simulink model "k1visetmy"  (Simulink 8.6)
settings: Solver=ode45  StartTime=0.0  StopTime=10.0  RelTol=1e-3
libraries: cdsCDI64 x10, cdsCDO64 x10, BIO_CD_DECODE_MASTER x10, BIO_CD_ENCODE_MASTER x9, cdsIPCx x5, dac x3, cdsEpicsOut x3, cdsBit2Word x2, cdsAdcx0 x1, cdsAdcx1 x1, cdsCDO32 x1, TYPEA_MASTER x1
settings Model: Creator=controls  LastModifiedBy=controls
settings DataIOCC: SignalLoggingSaveFormat=Dataset
settings OptimizationCC: ExpressionDepthLimit=128
settings DebuggingCC: UnderspecifiedInitializationDetection=Simplified  MergeDetectMultiDrivingBlocksExec=error  SolverPrmCheckMsg=none  FcnCallInpInsideContextMsg=EnableAllAsError  StateNameClashWarn=none
settings GRTTargetCC: CombineOutputUpdateFcns=on  GRTInterface=off

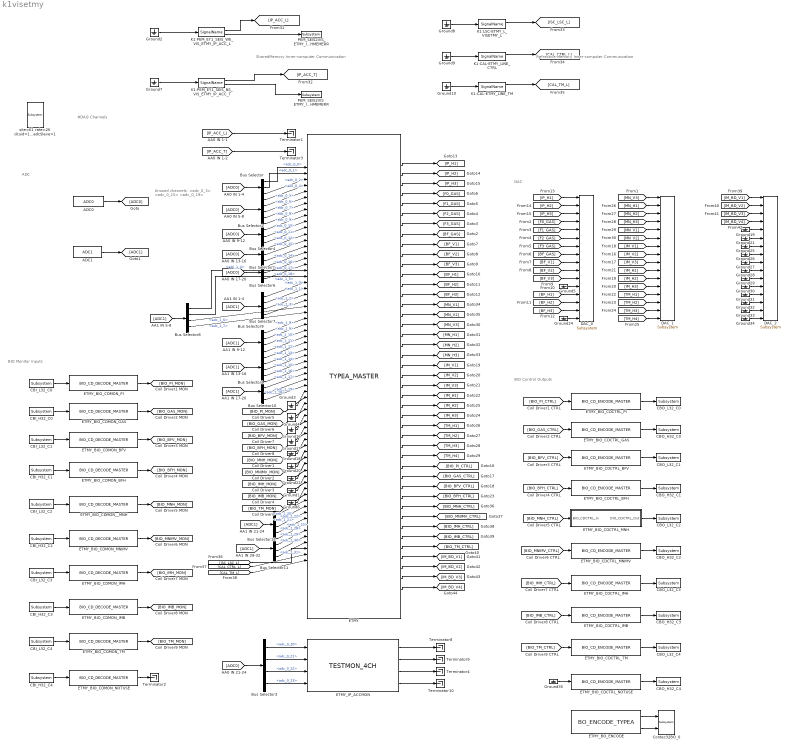
== system k1visetmy ==
  note: Unused channels:
      | <adc_0_3>
      | <adc_0_15>
      | <adc_0_19>
  note: #DAQ Channels
  note: BIO Monitor Inputs
  note: BIO Control Outputs
  note: DAC
  note: ADC
  note: SharedMemory
      | Inner-computer Communication
  note: Refrective Memory
      | Inner-computer Communication
  ADC0 : cdsAdcx0/ADC0  Tag=cdsAdc  Description=|
      | type-GSC_16AI64SSA
      | card_num=0
      settings: AttributesFormatString=%<Description>\n%<Tag>
  ADC1 : cdsAdcx1/ADC1  Tag=cdsAdc  Description=|
      | type-GSC_16AI64SSA
      | card_num=1
      settings: AttributesFormatString=%<Description>\n%<Tag>
  Bus Selector : BusSelector  OutputSignals=adc_0_0,adc_0_1,adc_0_2
  Bus Selector1 : BusSelector  OutputSignals=adc_1_12,adc_1_13,adc_1_14,adc_1_15
  Bus Selector10 : BusSelector  OutputSignals=adc_1_16,adc_1_17,adc_1_18,adc_1_19
  Bus Selector11 : BusSelector  OutputSignals=adc_1_28,adc_1_29,adc_1_30,adc_1_31
  Bus Selector12 : BusSelector  OutputSignals=adc_1_20,adc_1_21,adc_1_22,adc_1_23
  Bus Selector2 : BusSelector  OutputSignals=adc_0_4,adc_0_5,adc_0_6,adc_0_7
  Bus Selector3 : BusSelector  OutputSignals=adc_0_20,adc_0_21,adc_0_22,adc_0_23
  Bus Selector4 : BusSelector  OutputSignals=adc_0_8,adc_0_9,adc_0_10,adc_0_11
  Bus Selector5 : BusSelector  OutputSignals=adc_0_12,adc_0_15,adc_0_14
  Bus Selector6 : BusSelector  OutputSignals=adc_0_16,adc_0_17,adc_0_18
  Bus Selector7 : BusSelector  OutputSignals=adc_1_0,adc_1_1,adc_1_2,adc_1_3
  Bus Selector8 : BusSelector  OutputSignals=adc_1_4,adc_1_5,adc_1_6,adc_1_7
  Bus Selector9 : BusSelector  OutputSignals=adc_1_8,adc_1_9,adc_1_10,adc_1_11
  CBI_H32_C0 : cdsCDI64/Subsystem  Tag=cdsCDI64  Description=card_num=1
      settings: AttributesFormatString=%<Tag>\n%<Description>
  CBI_H32_C1 : cdsCDI64/Subsystem  Tag=cdsCDI64  Description=card_num=3
      settings: AttributesFormatString=%<Tag>\n%<Description>
  CBI_H32_C2 : cdsCDI64/Subsystem  Tag=cdsCDI64  Description=card_num=5
      settings: AttributesFormatString=%<Tag>\n%<Description>
  CBI_H32_C3 : cdsCDI64/Subsystem  Tag=cdsCDI64  Description=card_num=7
      settings: AttributesFormatString=%<Tag>\n%<Description>
  CBI_H32_C4 : cdsCDI64/Subsystem  Tag=cdsCDI64  Description=card_num=9
      settings: AttributesFormatString=%<Tag>\n%<Description>
  CBI_L32_C0 : cdsCDI64/Subsystem  Tag=cdsCDI64  Description=card_num=0
      settings: AttributesFormatString=%<Tag>\n%<Description>
  CBI_L32_C1 : cdsCDI64/Subsystem  Tag=cdsCDI64  Description=card_num=2
      settings: AttributesFormatString=%<Tag>\n%<Description>
  CBI_L32_C2 : cdsCDI64/Subsystem  Tag=cdsCDI64  Description=card_num=4
      settings: AttributesFormatString=%<Tag>\n%<Description>
  CBI_L32_C3 : cdsCDI64/Subsystem  Tag=cdsCDI64  Description=card_num=6
      settings: AttributesFormatString=%<Tag>\n%<Description>
  CBI_L32_C4 : cdsCDI64/Subsystem  Tag=cdsCDI64  Description=card_num=8
      settings: AttributesFormatString=%<Tag>\n%<Description>
  CBO_H32_C0 : cdsCDO64/Subsystem  Tag=cdsCDO64  Description=card_num=1
      settings: AttributesFormatString=%<Tag>\n%<Description>
  CBO_H32_C1 : cdsCDO64/Subsystem  Tag=cdsCDO64  Description=card_num=3
      settings: AttributesFormatString=%<Tag>\n%<Description>
  CBO_H32_C2 : cdsCDO64/Subsystem  Tag=cdsCDO64  Description=card_num=5
      settings: AttributesFormatString=%<Tag>\n%<Description>
  CBO_H32_C3 : cdsCDO64/Subsystem  Tag=cdsCDO64  Description=card_num=7
      settings: AttributesFormatString=%<Tag>\n%<Description>
  CBO_H32_C4 : cdsCDO64/Subsystem  Tag=cdsCDO64  Description=card_num=9
      settings: AttributesFormatString=%<Tag>\n%<Description>
  CBO_L32_C0 : cdsCDO64/Subsystem  Tag=cdsCDO64  Description=card_num=0
      settings: AttributesFormatString=%<Tag>\n%<Description>
  CBO_L32_C1 : cdsCDO64/Subsystem  Tag=cdsCDO64  Description=card_num=2
      settings: AttributesFormatString=%<Tag>\n%<Description>
  CBO_L32_C2 : cdsCDO64/Subsystem  Tag=cdsCDO64  Description=card_num=4
      settings: AttributesFormatString=%<Tag>\n%<Description>
  CBO_L32_C3 : cdsCDO64/Subsystem  Tag=cdsCDO64  Description=card_num=6
      settings: AttributesFormatString=%<Tag>\n%<Description>
  CBO_L32_C4 : cdsCDO64/Subsystem  Tag=cdsCDO64  Description=card_num=8
      settings: AttributesFormatString=%<Tag>\n%<Description>
  Contec32BO_0 : cdsCDO32/Subsystem  Tag=cdsCDO32  Description=Contec32 bit binary output module driver
      settings: AttributesFormatString=%<Tag>
  DAC_0 : dac/Subsystem  Description=|
      | type=GSC_16AO16,
      | card_num=0
      settings: AttributesFormatString=%<Description>
  DAC_1 : dac/Subsystem  Description=|
      | type=GSC_16AO16,
      | card_num=1
      settings: AttributesFormatString=%<Description>
  DAC_2 : dac/Subsystem  Description=|
      | type=GSC_16AO16,
      | card_num=2
      settings: AttributesFormatString=%<Description>
  ETMY : TYPEA_MASTER/TYPEA_MASTER
  ETMY_BIO_CDCTRL_BFH : BIO_CD_ENCODE_MASTER/BIO_CD_ENCODE_MASTER
  ETMY_BIO_CDCTRL_BFV : BIO_CD_ENCODE_MASTER/BIO_CD_ENCODE_MASTER
  ETMY_BIO_CDCTRL_GAS : BIO_CD_ENCODE_MASTER/BIO_CD_ENCODE_MASTER
  ETMY_BIO_CDCTRL_IMB : BIO_CD_ENCODE_MASTER/BIO_CD_ENCODE_MASTER
  ETMY_BIO_CDCTRL_IMH : BIO_CD_ENCODE_MASTER/BIO_CD_ENCODE_MASTER
  ETMY_BIO_CDCTRL_MNH : Subsystem
  ETMY_BIO_CDCTRL_MNIMV : BIO_CD_ENCODE_MASTER/BIO_CD_ENCODE_MASTER
  ETMY_BIO_CDCTRL_NOTUSE : BIO_CD_ENCODE_MASTER/BIO_CD_ENCODE_MASTER
  ETMY_BIO_CDCTRL_PI : BIO_CD_ENCODE_MASTER/BIO_CD_ENCODE_MASTER
  ETMY_BIO_CDCTRL_TM : BIO_CD_ENCODE_MASTER/BIO_CD_ENCODE_MASTER
  ETMY_BIO_CDMON_BFH : BIO_CD_DECODE_MASTER/BIO_CD_DECODE_MASTER
  ETMY_BIO_CDMON_BFV : BIO_CD_DECODE_MASTER/BIO_CD_DECODE_MASTER
  ETMY_BIO_CDMON_GAS : BIO_CD_DECODE_MASTER/BIO_CD_DECODE_MASTER
  ETMY_BIO_CDMON_IMB : BIO_CD_DECODE_MASTER/BIO_CD_DECODE_MASTER
  ETMY_BIO_CDMON_IMH : BIO_CD_DECODE_MASTER/BIO_CD_DECODE_MASTER
  ETMY_BIO_CDMON_MNIMV : BIO_CD_DECODE_MASTER/BIO_CD_DECODE_MASTER
  ETMY_BIO_CDMON_NOTUSE : BIO_CD_DECODE_MASTER/BIO_CD_DECODE_MASTER
  ETMY_BIO_CDMON_PI : BIO_CD_DECODE_MASTER/BIO_CD_DECODE_MASTER
  ETMY_BIO_CDMON_TM : BIO_CD_DECODE_MASTER/BIO_CD_DECODE_MASTER
  ETMY_BIO_CDMON__MNH : BIO_CD_DECODE_MASTER/BIO_CD_DECODE_MASTER
  ETMY_BO_ENCODE : BO_TYPEA_MASTER/BO_ENCODE_TYPEA
  ETMY_IP_ACCMON : TESTMON_4CH_MASTER/TESTMON_4CH
  Ground{1..10,16..22,24..35} (29 alike) : Ground
  K1:CAL-ETMY_LINE_CTRL : cdsIPCx/SignalName  Tag=cdsIPCx_RFM  Description=card=0
      settings: AttributesFormatString=%<Description>\n%<Tag>
  K1:CAL-ETMY_LINE_TM : cdsIPCx/SignalName  Tag=cdsIPCx_RFM  Description=card=0
      settings: AttributesFormatString=%<Description>\n%<Tag>
  K1:LSC-ETMY_L_VISETMY_L : cdsIPCx/SignalName  Tag=cdsIPCx_RFM  Description=card=0
      settings: AttributesFormatString=%<Description>\n%<Tag>
  K1:PEM_EY1_SEIS_NS_VIS_ETMY_IP_ACC_T : cdsIPCx/SignalName  Tag=cdsIPCx_SHMEM  Description=Inter-Process Communication via Shared memory.
      settings: AttributesFormatString=%<Tag>
  K1:PEM_EY1_SEIS_WE_VIS_ETMY_IP_ACC_L : cdsIPCx/SignalName  Tag=cdsIPCx_SHMEM  Description=Inter-Process Communication via Shared memory.
      settings: AttributesFormatString=%<Tag>
  PEM_SEIS2VIS_ETMY_IP_ACC_L_SHMEMERR : cdsEpicsOut/Subsystem  Tag=cdsEpicsOutput  Description=|
      | Purpose:                                          
      | Output a FE signal to an EPICS channel.           
      |                                                   
      | Operation:                                        
      | Takes input value and passes it to EPICS record.  
      |                                                   
      | Usage:                                            
      | Name the part with the desired EPICS rrecord name.
      settings: AttributesFormatString=%<Tag>
  PEM_SEIS2VIS_ETMY_IP_ACC_T_SHMEMERR : cdsEpicsOut/Subsystem  Tag=cdsEpicsOutput  Description=|
      | Purpose:                                          
      | Output a FE signal to an EPICS channel.           
      |                                                   
      | Operation:                                        
      | Takes input value and passes it to EPICS record.  
      |                                                   
      | Usage:                                            
      | Name the part with the desired EPICS rrecord name.
      settings: AttributesFormatString=%<Tag>
  Terminator{1..4,8..10} (7 alike) : Terminator
  site=K1 rate=2K dcuid=106 host=k1ey1 specific_cpu=3 adcSlave=1 : cdsParameters/Subsystem  Tag=cdsParameters  Description=|
      | Purpose:                                                                                                                                                                                                                                
      | Provide system parameters to the FE code generator to properly configure the generated EPICS names, rep rate of the FE controller, and the Data Acquisition node ID for proper storage of data from this FE controller.                 
      |                                                                                                                                                                                                                                         
      | Useage:                                                                                                                                                                                                                                 
      | The part NAME field is used to identify the FE parameters. It must be of the form:                                                                                                                                                      
      | site=                                                                                                                                                                                                                                   
      | rate=                                                                                                                                                                                                                                   
      | dcuid=                                                                                                                                                                                                                                  
      |                                                                                                                                                                                                                                         
      | Where:                                                                                                                                                                                                                                  
      | site= argument may be H1, H2, L1, M1, G1, either as a single argument or multiple, for example site=H1,H2. These are the only names allowed. These will become the first two characters of all EPICS and signal names (for example G1:).
      |                                                                                                                                                                                                                                         
      | rate= may be 2K, 16K, 32K, or 64K                                                                                                                                                                                                       
      |                                                                                                                                                                                                                                         
      | dcuid= is site specific ie it must be unique at each site.
      settings: AttributesFormatString=%<Tag>
  wires:
  ADC0/1 -> [ADC0]
  ADC1/1 -> [ADC1]
  [ADC0] -> Bus Selector/1
  [ADC0] -> Bus Selector2/1
  [ADC0] -> Bus Selector4/1
  [ADC0] -> Bus Selector5/1
  Bus Selector5/1 -> ETMY/12  "<adc_0_12>"
  Bus Selector5/3 -> ETMY/14  "<adc_0_14>"
  Bus Selector5/2 -> ETMY/13  "<adc_0_15>"
  [ADC0] -> Bus Selector6/1
  Bus Selector6/1 -> ETMY/15  "<adc_0_16>"
  Bus Selector6/2 -> ETMY/16  "<adc_0_17>"
  ETMY/10 -> [BF_V2]
  ETMY/11 -> [BF_V3]
  ETMY/12 -> [BF_H1]
  ETMY/13 -> [BF_H2]
  ETMY/14 -> [BF_H3]
  [BF_H2] -> DAC_0/14
  [BF_V3] -> DAC_0/11
  [BF_H3] -> DAC_0/15
  [BF_V1] -> DAC_0/9
  [BF_H1] -> DAC_0/13
  [BF_V2] -> DAC_0/10
  CBI_H32_C0/1 -> ETMY_BIO_CDMON_GAS/1
  CBI_L32_C1/1 -> ETMY_BIO_CDMON_BFV/1
  CBI_L32_C0/1 -> ETMY_BIO_CDMON_PI/1
  CBI_H32_C1/1 -> ETMY_BIO_CDMON_BFH/1
  ETMY_BIO_CDCTRL_BFH/1 -> CBO_H32_C1/1
  ETMY_BIO_CDCTRL_PI/1 -> CBO_L32_C0/1
  ETMY_BIO_CDCTRL_GAS/1 -> CBO_H32_C0/1
  ETMY_BIO_CDCTRL_BFV/1 -> CBO_L32_C1/1
  [BIO_PI_CTRL] -> ETMY_BIO_CDCTRL_PI/1
  [BIO_GAS_CTRL] -> ETMY_BIO_CDCTRL_GAS/1
  [BIO_BFV_CTRL] -> ETMY_BIO_CDCTRL_BFV/1
  ETMY_BIO_CDMON_PI/1 -> [BIO_PI_MON]
  ETMY_BIO_CDMON_GAS/1 -> [BIO_GAS_MON]
  ETMY_BIO_CDMON_BFH/1 -> [BIO_BFH_MON]
  ETMY_BIO_CDMON_BFV/1 -> [BIO_BFV_MON]
  [BIO_BFH_CTRL] -> ETMY_BIO_CDCTRL_BFH/1
  Bus Selector/1 -> ETMY/1  "<adc_0_0>"
  Bus Selector/2 -> ETMY/2  "<adc_0_1>"
  Bus Selector/3 -> ETMY/3  "<adc_0_2>"
  Bus Selector2/1 -> ETMY/4  "<adc_0_4>"
  Bus Selector2/2 -> ETMY/5  "<adc_0_5>"
  Bus Selector2/3 -> ETMY/6  "<adc_0_6>"
  Bus Selector2/4 -> ETMY/7  "<adc_0_7>"
  Bus Selector4/1 -> ETMY/8  "<adc_0_8>"
  Bus Selector4/2 -> ETMY/9  "<adc_0_9>"
  Bus Selector4/3 -> ETMY/10  "<adc_0_10>"
  Bus Selector4/4 -> ETMY/11  "<adc_0_11>"
  [IP_H1] -> DAC_0/1
  [IP_H2] -> DAC_0/2
  [IP_H3] -> DAC_0/3
  [F0_GAS] -> DAC_0/4
  [F1_GAS] -> DAC_0/5
  [F2_GAS] -> DAC_0/6
  [F3_GAS] -> DAC_0/7
  [BF_GAS] -> DAC_0/8
  [ADC0] -> Bus Selector3/1
  Bus Selector3/2 -> ETMY_IP_ACCMON/2  "<adc_0_21>"
  Bus Selector3/1 -> ETMY_IP_ACCMON/1  "<adc_0_20>"
  Bus Selector3/3 -> ETMY_IP_ACCMON/3  "<adc_0_22>"
  Bus Selector3/4 -> ETMY_IP_ACCMON/4  "<adc_0_23>"
  ETMY_IP_ACCMON/3 -> Terminator4/1
  ETMY_IP_ACCMON/4 -> Terminator10/1
  ETMY_IP_ACCMON/1 -> Terminator8/1
  ETMY_IP_ACCMON/2 -> Terminator9/1
  Bus Selector6/3 -> ETMY/17  "<adc_0_18>"
  Ground5/1 -> DAC_0/12
  Ground24/1 -> DAC_0/16
  [ADC1] -> Bus Selector7/1
  [ADC1] -> Bus Selector8/1
  [ADC1] -> Bus Selector9/1
  [IM_H2] -> DAC_1/11
  [IM_H1] -> DAC_1/10
  [IM_V1] -> DAC_1/7
  [IM_V2] -> DAC_1/8
  [IM_V3] -> DAC_1/9
  [TM_H3] -> DAC_1/15
  [TM_H2] -> DAC_1/14
  [TM_H1] -> DAC_1/13
  [TM_H4] -> DAC_1/16
  [IM_H3] -> DAC_1/12
  [MN_V3] -> DAC_1/1
  [MN_H1] -> DAC_1/2
  [MN_H2] -> DAC_1/3
  [MN_H3] -> DAC_1/4
  [MN_V1] -> DAC_1/5
  [MN_V2] -> DAC_1/6
  [ADC1] -> Bus Selector1/1
  [ADC1] -> Bus Selector10/1
  [BIO_PI_MON] -> ETMY/39
  [BIO_GAS_MON] -> ETMY/41
  [BIO_BFV_MON] -> ETMY/43
  [BIO_BFH_MON] -> ETMY/45
  Ground3/1 -> ETMY/38
  Ground4/1 -> ETMY/40
  Ground16/1 -> ETMY/42
  Ground17/1 -> ETMY/44
  Ground18/1 -> ETMY/46
  [BIO_MNH_MON] -> ETMY/47
  Ground20/1 -> ETMY/48
  [BIO_MNIMV_MON] -> ETMY/49
  Ground22/1 -> ETMY/50
  [BIO_IMH_MON] -> ETMY/51
  Bus Selector8/1 -> ETMY/18  "<adc_1_4>"
  Bus Selector8/2 -> ETMY/19  "<adc_1_5>"
  Bus Selector8/3 -> ETMY/24  "<adc_1_6>"
  Bus Selector8/4 -> ETMY/25  "<adc_1_7>"
  Bus Selector7/1 -> ETMY/20  "<adc_1_0>"
  Bus Selector7/2 -> ETMY/21  "<adc_1_1>"
  Bus Selector7/3 -> ETMY/22  "<adc_1_2>"
  Bus Selector7/4 -> ETMY/23  "<adc_1_3>"
  Bus Selector9/1 -> ETMY/26  "<adc_1_8>"
  Bus Selector9/2 -> ETMY/27  "<adc_1_9>"
  Bus Selector9/3 -> ETMY/28  "<adc_1_10>"
  Bus Selector9/4 -> ETMY/29  "<adc_1_11>"
  Bus Selector1/1 -> ETMY/30  "<adc_1_12>"
  Bus Selector1/2 -> ETMY/31  "<adc_1_13>"
  Bus Selector1/3 -> ETMY/32  "<adc_1_14>"
  Bus Selector1/4 -> ETMY/33  "<adc_1_15>"
  Bus Selector10/1 -> ETMY/34  "<adc_1_16>"
  Bus Selector10/2 -> ETMY/35  "<adc_1_17>"
  Bus Selector10/3 -> ETMY/36  "<adc_1_18>"
  Bus Selector10/4 -> ETMY/37  "<adc_1_19>"
  Ground1/1 -> ETMY/52
  Ground6/1 -> ETMY/54
  [BIO_IMB_MON] -> ETMY/53
  [BIO_TM_MON] -> ETMY/55
  ETMY/15 -> [MN_V1]
  ETMY/16 -> [MN_V2]
  ETMY/17 -> [MN_V3]
  ETMY/19 -> [MN_H2]
  ETMY/18 -> [MN_H1]
  ETMY/21 -> [IM_V1]
  ETMY/20 -> [MN_H3]
  ETMY/22 -> [IM_V2]
  ETMY/23 -> [IM_V3]
  ETMY/25 -> [IM_H2]
  ETMY/24 -> [IM_H1]
  ETMY/27 -> [TM_H1]
  ETMY/26 -> [IM_H3]
  ETMY/28 -> [TM_H2]
  ETMY/30 -> [TM_H4]
  ETMY/29 -> [TM_H3]
  ETMY/31 -> [BIO_PI_CTRL]
  ETMY/32 -> [BIO_GAS_CTRL]
  ETMY/33 -> [BIO_BFV_CTRL]
  ETMY/37 -> [BIO_IMH_CTRL]
  ETMY/34 -> [BIO_BFH_CTRL]
  ETMY/36 -> [BIO_MNIMV_CTRL]
  ETMY/35 -> [BIO_MNH_CTRL]
  ETMY/39 -> [BIO_TM_CTRL]
  ETMY/38 -> [BIO_IMB_CTRL]
  ETMY_BIO_CDCTRL_MNH/1(DIO_CDCTRL_Out) -> CBO_L32_C2/1
  ETMY_BIO_CDCTRL_MNIMV/1 -> CBO_H32_C2/1
  [BIO_MNH_CTRL] -> ETMY_BIO_CDCTRL_MNH/1(BIO_CDCTRL_In)
  [BIO_MNIMV_CTRL] -> ETMY_BIO_CDCTRL_MNIMV/1
  CBI_L32_C2/1 -> ETMY_BIO_CDMON__MNH/1
  CBI_H32_C2/1 -> ETMY_BIO_CDMON_MNIMV/1
  ETMY_BIO_CDMON__MNH/1 -> [BIO_MNH_MON]
  ETMY_BIO_CDMON_MNIMV/1 -> [BIO_MNIMV_MON]
  Ground19/1 -> DAC_2/5
  Ground21/1 -> DAC_2/6
  Ground25/1 -> DAC_2/7
  Ground26/1 -> DAC_2/8
  Ground27/1 -> DAC_2/9
  Ground28/1 -> DAC_2/10
  Ground29/1 -> DAC_2/11
  Ground30/1 -> DAC_2/12
  Ground31/1 -> DAC_2/13
  Ground32/1 -> DAC_2/14
  Ground33/1 -> DAC_2/15
  Ground34/1 -> DAC_2/16
  CBI_L32_C3/1 -> ETMY_BIO_CDMON_IMH/1
  CBI_H32_C3/1 -> ETMY_BIO_CDMON_IMB/1
  CBI_L32_C4/1 -> ETMY_BIO_CDMON_TM/1
  CBI_H32_C4/1 -> ETMY_BIO_CDMON_NOTUSE/1
  ETMY_BIO_CDCTRL_IMH/1 -> CBO_L32_C3/1
  ETMY_BIO_CDCTRL_IMB/1 -> CBO_H32_C3/1
  ETMY_BIO_CDCTRL_TM/1 -> CBO_L32_C4/1
  ETMY_BIO_CDCTRL_NOTUSE/1 -> CBO_H32_C4/1
  Ground35/1 -> ETMY_BIO_CDCTRL_NOTUSE/1
  ETMY_BIO_CDMON_NOTUSE/1 -> Terminator2/1
  ETMY_BIO_CDMON_TM/1 -> [BIO_TM_MON]
  ETMY_BIO_CDMON_IMB/1 -> [BIO_IMB_MON]
  ETMY_BIO_CDMON_IMH/1 -> [BIO_IMH_MON]
  [BIO_IMH_CTRL] -> ETMY_BIO_CDCTRL_IMH/1
  [BIO_TM_CTRL] -> ETMY_BIO_CDCTRL_TM/1
  [BIO_IMB_CTRL] -> ETMY_BIO_CDCTRL_IMB/1
  [IM_BD_V1] -> DAC_2/1
  [IM_BD_V3] -> DAC_2/3
  ETMY_BO_ENCODE/1 -> Contec32BO_0/1
  ETMY_BO_ENCODE/2 -> Contec32BO_0/2
  [ADC1] -> Bus Selector11/1
  Bus Selector11/1 -> ETMY/60  "<adc_1_28>"
  Bus Selector11/2 -> ETMY/61  "<adc_1_29>"
  Bus Selector11/3 -> ETMY/62  "<adc_1_30>"
  Bus Selector11/4 -> ETMY/63  "<adc_1_31>"
  [ADC1] -> Bus Selector12/1
  Bus Selector12/1 -> ETMY/56  "<adc_1_20>"
  Bus Selector12/2 -> ETMY/57  "<adc_1_21>"
  Bus Selector12/3 -> ETMY/58  "<adc_1_22>"
  Bus Selector12/4 -> ETMY/59  "<adc_1_23>"
  Ground2/1 -> K1:PEM_EY1_SEIS_WE_VIS_ETMY_IP_ACC_L/1
  K1:PEM_EY1_SEIS_WE_VIS_ETMY_IP_ACC_L/2 -> PEM_SEIS2VIS_ETMY_IP_ACC_L_SHMEMERR/1
  K1:PEM_EY1_SEIS_WE_VIS_ETMY_IP_ACC_L/1 -> [IP_ACC_L]
  K1:PEM_EY1_SEIS_NS_VIS_ETMY_IP_ACC_T/1 -> [IP_ACC_T]
  K1:PEM_EY1_SEIS_NS_VIS_ETMY_IP_ACC_T/2 -> PEM_SEIS2VIS_ETMY_IP_ACC_T_SHMEMERR/1
  Ground7/1 -> K1:PEM_EY1_SEIS_NS_VIS_ETMY_IP_ACC_T/1
  [IP_ACC_T] -> Terminator3/1
  [IP_ACC_L] -> Terminator1/1
  Ground8/1 -> K1:LSC-ETMY_L_VISETMY_L/1
  K1:LSC-ETMY_L_VISETMY_L/1 -> [ISC_LSC_L]
  K1:CAL-ETMY_LINE_CTRL/1 -> [CAL_CTRL_L]
  Ground9/1 -> K1:CAL-ETMY_LINE_CTRL/1
  K1:CAL-ETMY_LINE_TM/1 -> [CAL_TM_L]
  Ground10/1 -> K1:CAL-ETMY_LINE_TM/1
  [CAL_CTRL_L] -> ETMY/65
  [CAL_TM_L] -> ETMY/66
  ETMY/1 -> [IP_H1]
  ETMY/2 -> [IP_H2]
  ETMY/3 -> [IP_H3]
  ETMY/4 -> [F0_GAS]
  ETMY/5 -> [F1_GAS]
  ETMY/6 -> [F2_GAS]
  ETMY/7 -> [F3_GAS]
  ETMY/8 -> [BF_GAS]
  ETMY/9 -> [BF_V1]
  ETMY/40 -> [IM_BD_V1]
  ETMY/41 -> [IM_BD_V2]
  ETMY/42 -> [IM_BD_V3]
  ETMY/43 -> [IM_BD_V4]
  [IM_BD_V2] -> DAC_2/2
  [IM_BD_V4] -> DAC_2/4
  [ISC_LSC_L] -> ETMY/64

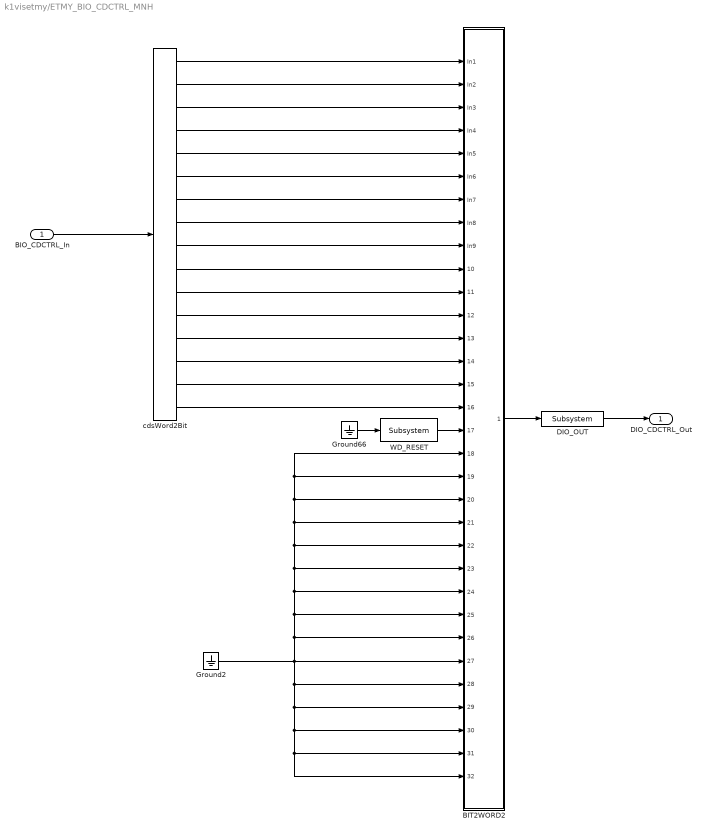
== system k1visetmy/ETMY_BIO_CDCTRL_MNH ==
  BIO_CDCTRL_In : Inport
  BIT2WORD2 : Subsystem
  DIO_OUT : cdsEpicsOut/Subsystem  Tag=cdsEpicsOutput  Description=|
      | Purpose:                                          
      | Output a FE signal to an EPICS channel.           
      |                                                   
      | Operation:                                        
      | Takes input value and passes it to EPICS record.  
      |                                                   
      | Usage:                                            
      | Name the part with the desired EPICS rrecord name.
      settings: AttributesFormatString=%<Tag>
  Ground2 : Ground
  Ground66 : Ground
  WD_RESET : cdsEpicsBinIn/Subsystem  Tag=cdsEpicsBinIn  Description=|
      | Purpose:                                                                            
      | Create an EPICS binary (0 or 1) input channel to the FE realtime controls.          
      |                                                                                     
      | Operation:                                                                          
      | Outputs value from an EPICS ai record. Value is binary input (bi Epics record type).
      |                                                                                     
      | Usage:                                                                              
      | Name the part with the desired EPICS channel name.
      settings: AttributesFormatString=%<Tag>
  cdsWord2Bit : cdsWord2Bit/cdsWord2Bit  Tag=cdsWord2Bit  Description=Generate 16 0/1 outputs from single 16-bit integer input
      settings: AttributesFormatString=cdsWord2Bit
  DIO_CDCTRL_Out : Outport
  wires:
  BIT2WORD2/1(Out1) -> DIO_OUT/1
  DIO_OUT/1 -> DIO_CDCTRL_Out/1
  BIO_CDCTRL_In/1 -> cdsWord2Bit/1
  cdsWord2Bit/1 -> BIT2WORD2/1(In1)
  cdsWord2Bit/2 -> BIT2WORD2/2(In2)
  cdsWord2Bit/3 -> BIT2WORD2/3(In3)
  cdsWord2Bit/4 -> BIT2WORD2/4(In4)
  cdsWord2Bit/5 -> BIT2WORD2/5(In5)
  cdsWord2Bit/6 -> BIT2WORD2/6(In6)
  cdsWord2Bit/7 -> BIT2WORD2/7(In7)
  cdsWord2Bit/8 -> BIT2WORD2/8(In8)
  cdsWord2Bit/9 -> BIT2WORD2/9(In9)
  cdsWord2Bit/10 -> BIT2WORD2/10(In10)
  cdsWord2Bit/11 -> BIT2WORD2/11(In11)
  cdsWord2Bit/12 -> BIT2WORD2/12(In12)
  cdsWord2Bit/13 -> BIT2WORD2/13(In13)
  cdsWord2Bit/14 -> BIT2WORD2/14(In14)
  cdsWord2Bit/15 -> BIT2WORD2/15(In15)
  cdsWord2Bit/16 -> BIT2WORD2/16(In16)
  WD_RESET/1 -> BIT2WORD2/17(In17)
  Ground66/1 -> WD_RESET/1
  Ground2/1 -> BIT2WORD2/27(In27), BIT2WORD2/28(In28), BIT2WORD2/29(In29), BIT2WORD2/30(In30), BIT2WORD2/31(In31), BIT2WORD2/32(In32), BIT2WORD2/26(In26), BIT2WORD2/25(In25), BIT2WORD2/24(In24), BIT2WORD2/23(In23), BIT2WORD2/22(In22), BIT2WORD2/21(In21), BIT2WORD2/20(In20), BIT2WORD2/18(In18), BIT2WORD2/19(In19)

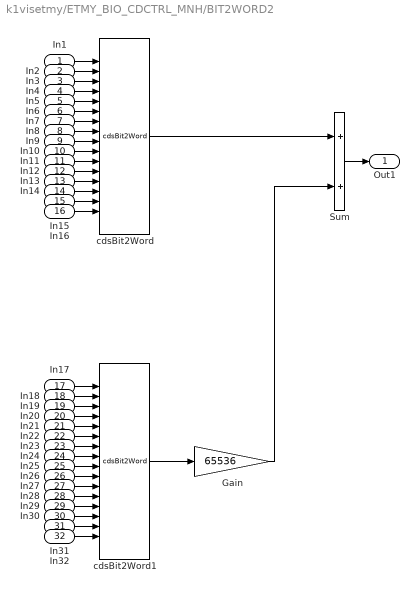
== system k1visetmy/ETMY_BIO_CDCTRL_MNH/BIT2WORD2 ==
  In1 : Inport
  In2 : Inport  Port=2
  In3 : Inport  Port=3
  In4 : Inport  Port=4
  In5 : Inport  Port=5
  In6 : Inport  Port=6
  In7 : Inport  Port=7
  In8 : Inport  Port=8
  In9 : Inport  Port=9
  In10 : Inport  Port=10
  In11 : Inport  Port=11
  In12 : Inport  Port=12
  In13 : Inport  Port=13
  In14 : Inport  Port=14
  In15 : Inport  Port=15
  In16 : Inport  Port=16
  In17 : Inport  Port=17
  In18 : Inport  Port=18
  In19 : Inport  Port=19
  In20 : Inport  Port=20
  In21 : Inport  Port=21
  In22 : Inport  Port=22
  In23 : Inport  Port=23
  In24 : Inport  Port=24
  In25 : Inport  Port=25
  In26 : Inport  Port=26
  In27 : Inport  Port=27
  In28 : Inport  Port=28
  In29 : Inport  Port=29
  In30 : Inport  Port=30
  In31 : Inport  Port=31
  In32 : Inport  Port=32
  Gain : Gain  Gain=65536
  Sum : Sum
  cdsBit2Word : cdsBit2Word/cdsBit2Word  Tag=cdsBit2Word  Description=Forms single 16 bit integer from 16 0/1 inputs.
      settings: AttributesFormatString=%<Tag>
  cdsBit2Word1 : cdsBit2Word/cdsBit2Word  Tag=cdsBit2Word  Description=Forms single 16 bit integer from 16 0/1 inputs.
      settings: AttributesFormatString=%<Tag>
  Out1 : Outport
  wires:
  In32/1 -> cdsBit2Word1/16
  In31/1 -> cdsBit2Word1/15
  In30/1 -> cdsBit2Word1/14
  In29/1 -> cdsBit2Word1/13
  In28/1 -> cdsBit2Word1/12
  In27/1 -> cdsBit2Word1/11
  In26/1 -> cdsBit2Word1/10
  In25/1 -> cdsBit2Word1/9
  In24/1 -> cdsBit2Word1/8
  In23/1 -> cdsBit2Word1/7
  In22/1 -> cdsBit2Word1/6
  In21/1 -> cdsBit2Word1/5
  In20/1 -> cdsBit2Word1/4
  In19/1 -> cdsBit2Word1/3
  In18/1 -> cdsBit2Word1/2
  In17/1 -> cdsBit2Word1/1
  In16/1 -> cdsBit2Word/16
  In15/1 -> cdsBit2Word/15
  In14/1 -> cdsBit2Word/14
  In13/1 -> cdsBit2Word/13
  In12/1 -> cdsBit2Word/12
  In11/1 -> cdsBit2Word/11
  Sum/1 -> Out1/1
  In10/1 -> cdsBit2Word/10
  In9/1 -> cdsBit2Word/9
  In8/1 -> cdsBit2Word/8
  In7/1 -> cdsBit2Word/7
  In6/1 -> cdsBit2Word/6
  In5/1 -> cdsBit2Word/5
  In4/1 -> cdsBit2Word/4
  In3/1 -> cdsBit2Word/3
  In2/1 -> cdsBit2Word/2
  In1/1 -> cdsBit2Word/1
  cdsBit2Word/1 -> Sum/1
  cdsBit2Word1/1 -> Gain/1
  Gain/1 -> Sum/2
